simulink model "w2_warplab_buffers"  (Simulink 7.7)
settings: Solver=VariableStepDiscrete  SolverMode=SingleTasking  StartTime=0.0  StopTime=200000  RelTol=1e-3
InitFcn:
  | w2_warplab_buffers_init
StartFcn:
  | w2_warplab_buffers_init
values from neighbouring files (symbols this model uses):
  NumSamps_Rx_IQ = 2^14    (= 16384)    [w2_warplab_buffers_init.m]
  NumSamps_Rx_RSSI = 2^12    (= 4096)    [w2_warplab_buffers_init.m]
  NumSamps_Tx_IQ = 2^14    (= 16384)    [w2_warplab_buffers_init.m]
undefined symbols (not defined in the file or in its folder): gcbh, xlBlockLoadCallback, xlGetNormalizedPeriod
libraries: xbsIndex_r4 x752
(part 5 of 7)

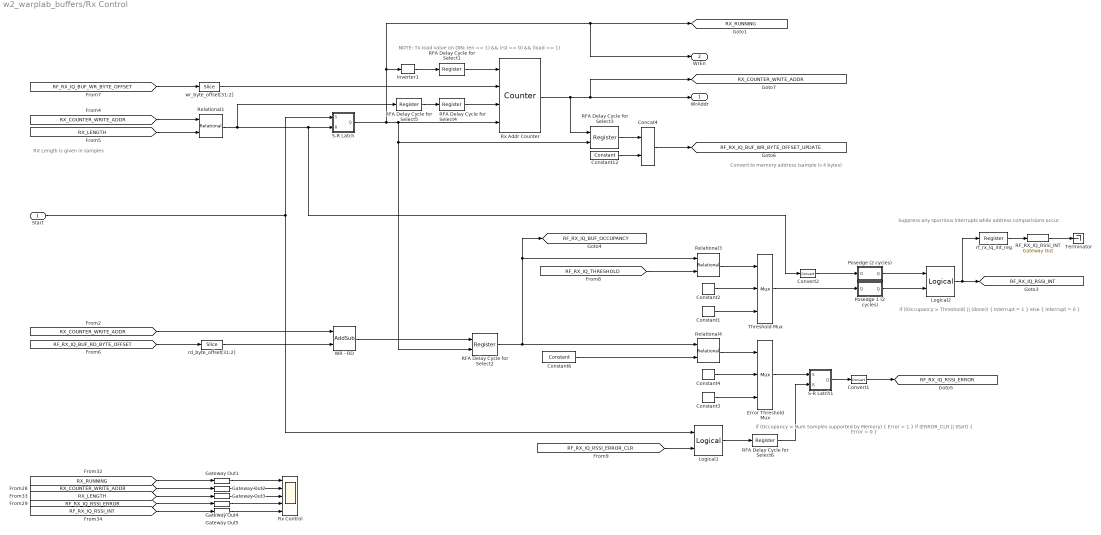
== system w2_warplab_buffers/Rx Control ==
  note: if ((Occupancy > Threshold) || (done)) {
      |     Interrupt = 1
      | } else {
      |     Interrupt = 0
      | }
  note: NOTE: To load value on DIN: (en == 1) && (rst == 0) && (load == 1)
  note: if (Occupancy > Num Samples supported by Memory) {
      |     Error = 1
      | }
      |
      | if (ERROR_CLR || Start) {
      |     Error = 0
      | }
  note: RX Length is given in samples
  note: Convert to memory address (sample is 4 bytes)
  note: Suppress any spurrious interrupts while
      | address comparisions occur.
  Start : Inport
  Concat4 : xbsIndex_r4/Concat  num_inputs=2  dbl_ovrd=off  block_type=concat
  Constant1 : xbsIndex_r4/Constant  const=1  gui_display_data_type=Fixed-point  arith_type=Unsigned  n_bits=1  bin_pt=0  preci_type=Single  exp_width=8  frac_width=24  explicit_period=off  period=1  equ=P=C  opselect=C  inp2=PCIN>>17  opr=+  inp1=P  carry=CIN  dbl_ovrd=off  block_type=constant
      settings: block_version=10.1.2
  Constant12 : xbsIndex_r4/Constant  const=0  gui_display_data_type=Fixed-point  arith_type=Unsigned  n_bits=2  bin_pt=0  preci_type=Single  exp_width=8  frac_width=24  explicit_period=off  period=1  equ=P=C  opselect=C  inp2=PCIN>>17  opr=+  inp1=P  carry=CIN  dbl_ovrd=off  block_type=constant
  Constant2 : xbsIndex_r4/Constant  const=0  gui_display_data_type=Fixed-point  arith_type=Unsigned  n_bits=1  bin_pt=0  preci_type=Single  exp_width=8  frac_width=24  explicit_period=off  period=1  equ=P=C  opselect=C  inp2=PCIN>>17  opr=+  inp1=P  carry=CIN  dbl_ovrd=off  block_type=constant
      settings: block_version=10.1.2
  Constant3 : xbsIndex_r4/Constant  const=1  gui_display_data_type=Fixed-point  arith_type=Unsigned  n_bits=1  bin_pt=0  preci_type=Single  exp_width=8  frac_width=24  explicit_period=off  period=1  equ=P=C  opselect=C  inp2=PCIN>>17  opr=+  inp1=P  carry=CIN  dbl_ovrd=off  block_type=constant
      settings: block_version=10.1.2
  Constant4 : xbsIndex_r4/Constant  const=0  gui_display_data_type=Fixed-point  arith_type=Unsigned  n_bits=1  bin_pt=0  preci_type=Single  exp_width=8  frac_width=24  explicit_period=off  period=1  equ=P=C  opselect=C  inp2=PCIN>>17  opr=+  inp1=P  carry=CIN  dbl_ovrd=off  block_type=constant
      settings: block_version=10.1.2
  Constant6 : xbsIndex_r4/Constant  const=NumSamps_Rx_IQ  gui_display_data_type=Fixed-point  arith_type=Unsigned  n_bits=30  bin_pt=0  preci_type=Single  exp_width=8  frac_width=24  explicit_period=off  period=1  equ=P=C  opselect=C  inp2=PCIN>>17  opr=+  inp1=P  carry=CIN  dbl_ovrd=off  block_type=constant
      settings: block_version=10.1.2
  Convert1 : xbsIndex_r4/Convert  gui_display_data_type=Fixed-point  arith_type=Unsigned  n_bits=1  bin_pt=0  float_type=Single  exp_bits=8  fraction_bits=24  quantization=Truncate  overflow=Wrap  en=off  latency=0  dbl_ovrd=off  pipeline=off  block_type=convert
      settings: block_version=10.1.2
  Convert2 : xbsIndex_r4/Convert  gui_display_data_type=Fixed-point  arith_type=Unsigned  n_bits=1  bin_pt=0  float_type=Single  exp_bits=8  fraction_bits=24  quantization=Truncate  overflow=Wrap  en=off  latency=0  dbl_ovrd=off  pipeline=off  block_type=convert
      settings: block_version=10.1.2
  Error Threshold Mux : xbsIndex_r4/Mux  inputs=2  en=off  latency=0  precision=Full  arith_type=Unsigned  n_bits=16  bin_pt=14  quantization=Truncate  overflow=Wrap  dbl_ovrd=off  block_type=mux
  Gateway Out{1..5} (5 alike) : xbsIndex_r4/Gateway Out  inherit_from_input=off  hdl_port=off  timing_constraint=None  locs_specified=off  LOCs={}  UseAsDAC=off  DACChannel='1'  block_type=gatewayout
      settings: infoedit="Gateway out block.  Converts Xilinx fixed point inputs into ouputs of type Simulink integer, double, or fixed point.<P><P>Hardware notes:  In hardware these blocks become top level output ports or are discarded, depending on how they are configured."  block_version=10.1.2
  Inverter1 : xbsIndex_r4/Inverter  en=off  latency=0  dbl_ovrd=off  block_type=inv
      settings: block_version=8.2
  Logical1 : xbsIndex_r4/Logical  logical_function=OR  inputs=2  en=off  latency=0  precision=Full  arith_type=Unsigned  n_bits=16  bin_pt=0  align_bp=on  dbl_ovrd=off  block_type=logical
  Logical2 : xbsIndex_r4/Logical  logical_function=OR  inputs=2  en=off  latency=0  precision=Full  arith_type=Unsigned  n_bits=16  bin_pt=0  align_bp=on  dbl_ovrd=off  block_type=logical
  Posedge (2 cycles) : Subsystem
  Posedge 1 (2 cycles) : Subsystem
  RFA Delay Cycle for Select{1,4..6} (4 alike) : xbsIndex_r4/Register  init=0  rst=off  en=off  dbl_ovrd=off  block_type=register
  RFA Delay Cycle for Select2 : xbsIndex_r4/Register  init=0  rst=off  en=on  dbl_ovrd=off  block_type=register
  RFA Delay Cycle for Select3 : xbsIndex_r4/Register  init=0  rst=off  en=on  dbl_ovrd=off  block_type=register
  RF_RX_IQ_RSSI_INT : xbsIndex_r4/Gateway Out  inherit_from_input=off  hdl_port=on  timing_constraint=None  locs_specified=off  LOCs={}  UseAsDAC=off  DACChannel='1'  block_type=gatewayout
      settings: block_version=8.2
  Relational1 : xbsIndex_r4/Relational  mode=a>=b  en=off  latency=0  dbl_ovrd=off  block_type=relational
      settings: block_version=8.2
  Relational3 : xbsIndex_r4/Relational  mode=a>b  en=off  latency=0  dbl_ovrd=off  block_type=relational
      settings: block_version=8.2
  Relational4 : xbsIndex_r4/Relational  mode=a>b  en=off  latency=0  dbl_ovrd=off  block_type=relational
      settings: block_version=8.2
  Rx Addr Counter : xbsIndex_r4/Counter  cnt_type=Free Running  cnt_to=Inf  operation=Up  start_count=0  cnt_by_val=1  arith_type=Unsigned  n_bits=30  bin_pt=0  load_pin=on  rst=on  en=on  explicit_period=off  period=1  dbl_ovrd=off  use_behavioral_HDL=off  implementation=Fabric  use_rpm=off  block_type=counter
      settings: block_version=8.2
  Rx Control : Scope  NumInputPorts=5
      settings: TimeRange=70000  YMin=0~0~0~0~0  YMax=1~1~1~100~20000
  S-R Latch : Subsystem
  S-R Latch1 : Subsystem
  Terminator : Terminator
  Threshold Mux : xbsIndex_r4/Mux  inputs=2  en=off  latency=0  precision=Full  arith_type=Unsigned  n_bits=16  bin_pt=14  quantization=Truncate  overflow=Wrap  dbl_ovrd=off  block_type=mux
  WR - RD : xbsIndex_r4/AddSub  mode=Subtraction  use_carryin=off  use_carryout=off  en=off  latency=0  precision=User Defined  arith_type=Unsigned  n_bits=30  bin_pt=0  quantization=Truncate  overflow=Wrap  dbl_ovrd=off  use_behavioral_HDL=off  hw_selection=Fabric  pipelined=off  block_type=addsub
  rd_byte_offset[31:2] : xbsIndex_r4/Slice  nbits=30  boolean_output=off  mode=Lower Bit Location + Width  bit1=0  base1=MSB of Input  bit0=2  base0=LSB of Input  dbl_ovrd=off  block_type=slice
  rf_rx_iq_int_reg : xbsIndex_r4/Register  init=0  rst=off  en=off  dbl_ovrd=off  block_type=register
  wr_byte_offset[31:2] : xbsIndex_r4/Slice  nbits=30  boolean_output=off  mode=Lower Bit Location + Width  bit1=0  base1=MSB of Input  bit0=2  base0=LSB of Input  dbl_ovrd=off  block_type=slice
  WrAddr : Outport
  WrEn : Outport  Port=2
  tag scope: RF_RX_IQ_BUF_OCCUPANCY=global, RF_RX_IQ_BUF_WR_BYTE_OFFSET_UPDATE=global, RF_RX_IQ_RSSI_ERROR=global, RF_RX_IQ_RSSI_INT=global, RX_COUNTER_WRITE_ADDR=global, RX_RUNNING=global
  wires:
  S-R Latch/1(Q) -> Inverter1/1, WrEn/1, [RX_RUNNING], Rx Addr Counter/4, RFA Delay Cycle for Select3/2, RFA Delay Cycle for Select2/2
  Gateway Out5/1 -> Rx Control/5
  Gateway Out4/1 -> Rx Control/4
  Gateway Out3/1 -> Rx Control/3
  Gateway Out2/1 -> Rx Control/2
  Gateway Out1/1 -> Rx Control/1
  [RF_RX_IQ_BUF_RD_BYTE_OFFSET] -> rd_byte_offset[31:2]/1
  Relational3/1 -> Threshold Mux/1
  Constant1/1 -> Threshold Mux/3
  Constant2/1 -> Threshold Mux/2
  [RF_RX_IQ_THRESHOLD] -> Relational3/2
  Relational4/1 -> Error Threshold Mux/1
  Constant3/1 -> Error Threshold Mux/3
  Constant4/1 -> Error Threshold Mux/2
  Error Threshold Mux/1 -> S-R Latch1/1(S)
  Constant6/1 -> Relational4/2
  [RX_LENGTH] -> Relational1/2
  Relational1/1 -> RFA Delay Cycle for Select5/1, S-R Latch/2(R), Convert2/1
  Rx Addr Counter/1 -> [RX_COUNTER_WRITE_ADDR], WrAddr/1, RFA Delay Cycle for Select3/1
  Constant12/1 -> Concat4/2
  Concat4/1 -> [RF_RX_IQ_BUF_WR_BYTE_OFFSET_UPDATE]
  S-R Latch1/1(Q) -> Convert1/1
  Convert1/1 -> [RF_RX_IQ_RSSI_ERROR]
  [RF_RX_IQ_BUF_WR_BYTE_OFFSET] -> wr_byte_offset[31:2]/1
  wr_byte_offset[31:2]/1 -> Rx Addr Counter/2
  Inverter1/1 -> RFA Delay Cycle for Select1/1
  RFA Delay Cycle for Select1/1 -> Rx Addr Counter/1
  RF_RX_IQ_RSSI_INT/1 -> Terminator/1
  Logical1/1 -> RFA Delay Cycle for Select6/1
  [RF_RX_IQ_RSSI_ERROR_CLR] -> Logical1/2
  RFA Delay Cycle for Select3/1 -> Concat4/1
  RFA Delay Cycle for Select4/1 -> Rx Addr Counter/3
  RFA Delay Cycle for Select5/1 -> RFA Delay Cycle for Select4/1
  Logical2/1 -> [RF_RX_IQ_RSSI_INT], rf_rx_iq_int_reg/1
  Threshold Mux/1 -> Posedge 1 (2 cycles)/1(D)
  Convert2/1 -> Posedge (2 cycles)/1(D)
  [RX_COUNTER_WRITE_ADDR] -> Relational1/1
  [RX_COUNTER_WRITE_ADDR] -> WR - RD/1
  rd_byte_offset[31:2]/1 -> WR - RD/2
  WR - RD/1 -> RFA Delay Cycle for Select2/1
  RFA Delay Cycle for Select2/1 -> Relational4/1, [RF_RX_IQ_BUF_OCCUPANCY], Relational3/1
  Start/1 -> S-R Latch/1(S), Logical1/1
  RFA Delay Cycle for Select6/1 -> S-R Latch1/2(R)
  [RX_RUNNING] -> Gateway Out1/1
  [RX_COUNTER_WRITE_ADDR] -> Gateway Out2/1
  [RX_LENGTH] -> Gateway Out3/1
  [RF_RX_IQ_RSSI_ERROR] -> Gateway Out4/1
  [RF_RX_IQ_RSSI_INT] -> Gateway Out5/1
  Posedge 1 (2 cycles)/1(Q) -> Logical2/2
  Posedge (2 cycles)/1(Q) -> Logical2/1
  rf_rx_iq_int_reg/1 -> RF_RX_IQ_RSSI_INT/1

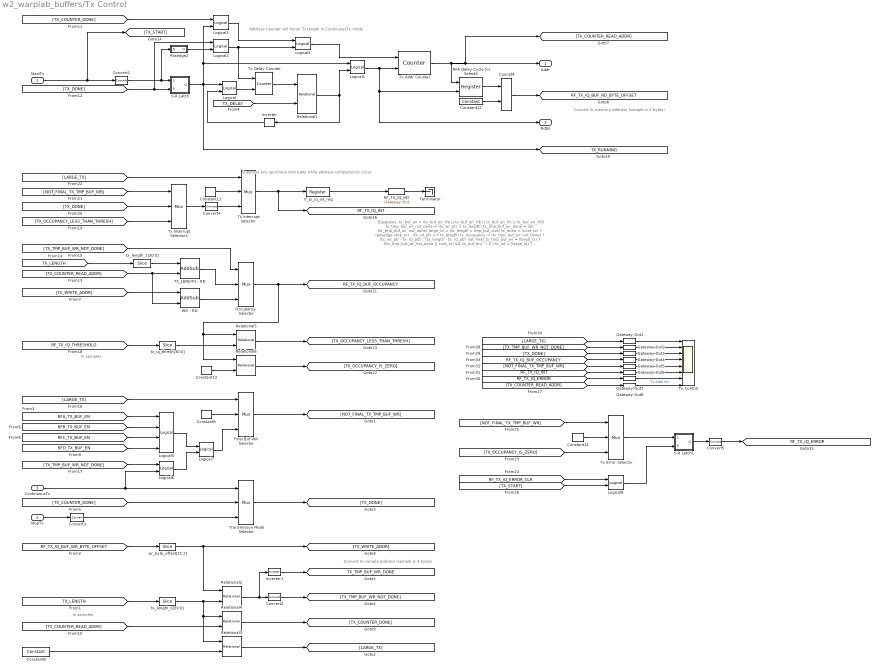
== system w2_warplab_buffers/Tx Control ==
  note: Address Counter will honor TxLength in ContinuousTx mode
  note: Convert to memory address (sample is 4 bytes)
  note: Convert to sample address (sample is 4 bytes)
  note: Equations:
      |   tx_buf_en               = (tx_buf_en_rfa || tx_buf_en_rfb || tx_buf_en_rfc || tx_buf_en_rfd)
      |
      |   tx_tmp_buf_wr_not_done  = (tx_wr_ptr < tx_length)
      |
      |   tx_tmp_buf_wr_done      = not (tx_tmp_buf_wr_not_done)
      |
      |   large_tx                = (tx_length > tmp_buf_size)
      |
      |   tx_done                 = (cont_tx) ? (posedge stop_tx) : (tx_rd_ptr >= tx_length)
      |
      |   tx_occupancy            = (tx_tmp_buf_wr_not_done) ? (tx_wr_ptr - tx_rd_ptr) : (tx_length - tx_rd_ptr)
      |
      |   not_final_tx_tmp_buf_wr = (large_tx) ? ((tx_tmp_buf_wr_not_done || cont_tx) && tx_buf_en) : ( 0 )
      |
      |   tx_int                  = (large_tx) ? ((not_final_tx_tmp_buf_wr) ? (tx_occupancy < tx_threshold) : tx_done) : ( 0 )
      |
      |   tx_err                  = (not_final_tx_tmp_buf_wr) ? (tx_occupancy == 0) : (0)
  note: In samples
  note: In samples
  note: Suppress any spurrious interrupts while
      | address comparisions occur.
  StartTx : Inport
  StopTx : Inport  Port=2
  ContinuousTx : Inport  Port=3
  Concat4 : xbsIndex_r4/Concat  num_inputs=2  dbl_ovrd=off  block_type=concat
  Constant11 : xbsIndex_r4/Constant  const=0  gui_display_data_type=Fixed-point  arith_type=Unsigned  n_bits=1  bin_pt=0  preci_type=Single  exp_width=8  frac_width=24  explicit_period=off  period=1  equ=P=C  opselect=C  inp2=PCIN>>17  opr=+  inp1=P  carry=CIN  dbl_ovrd=off  block_type=constant
      settings: block_version=10.1.2
  Constant12 : xbsIndex_r4/Constant  const=0  gui_display_data_type=Fixed-point  arith_type=Unsigned  n_bits=2  bin_pt=0  preci_type=Single  exp_width=8  frac_width=24  explicit_period=off  period=1  equ=P=C  opselect=C  inp2=PCIN>>17  opr=+  inp1=P  carry=CIN  dbl_ovrd=off  block_type=constant
  Constant13 : xbsIndex_r4/Constant  const=0  gui_display_data_type=Fixed-point  arith_type=Unsigned  n_bits=30  bin_pt=0  preci_type=Single  exp_width=8  frac_width=24  explicit_period=off  period=1  equ=P=C  opselect=C  inp2=PCIN>>17  opr=+  inp1=P  carry=CIN  dbl_ovrd=off  block_type=constant
      settings: block_version=10.1.2
  Constant14 : xbsIndex_r4/Constant  const=0  gui_display_data_type=Boolean  arith_type=Boolean  n_bits=1  bin_pt=0  preci_type=Single  exp_width=8  frac_width=24  explicit_period=off  period=1  equ=P=C  opselect=C  inp2=PCIN>>17  opr=+  inp1=P  carry=CIN  dbl_ovrd=off  block_type=constant
      settings: block_version=10.1.2
  Constant8 : xbsIndex_r4/Constant  const=NumSamps_Tx_IQ  gui_display_data_type=Fixed-point  arith_type=Unsigned  n_bits=30  bin_pt=0  preci_type=Single  exp_width=8  frac_width=24  explicit_period=off  period=1  equ=P=C  opselect=C  inp2=PCIN>>17  opr=+  inp1=P  carry=CIN  dbl_ovrd=off  block_type=constant
      settings: block_version=10.1.2
  Constant9 : xbsIndex_r4/Constant  const=0  gui_display_data_type=Fixed-point  arith_type=Unsigned  n_bits=1  bin_pt=0  preci_type=Single  exp_width=8  frac_width=24  explicit_period=off  period=1  equ=P=C  opselect=C  inp2=PCIN>>17  opr=+  inp1=P  carry=CIN  dbl_ovrd=off  block_type=constant
      settings: block_version=10.1.2
  Convert1 : xbsIndex_r4/Convert  gui_display_data_type=Fixed-point  arith_type=Boolean  n_bits=1  bin_pt=0  float_type=Single  exp_bits=8  fraction_bits=24  quantization=Truncate  overflow=Wrap  en=off  latency=0  dbl_ovrd=off  pipeline=off  block_type=convert
  Convert2 : xbsIndex_r4/Convert  gui_display_data_type=Fixed-point  arith_type=Unsigned  n_bits=1  bin_pt=0  float_type=Single  exp_bits=8  fraction_bits=24  quantization=Truncate  overflow=Wrap  en=off  latency=0  dbl_ovrd=off  pipeline=off  block_type=convert
  Convert3 : xbsIndex_r4/Convert  gui_display_data_type=Fixed-point  arith_type=Boolean  n_bits=1  bin_pt=0  float_type=Single  exp_bits=8  fraction_bits=24  quantization=Truncate  overflow=Wrap  en=off  latency=0  dbl_ovrd=off  pipeline=off  block_type=convert
  Convert4 : xbsIndex_r4/Convert  gui_display_data_type=Fixed-point  arith_type=Unsigned  n_bits=1  bin_pt=0  float_type=Single  exp_bits=8  fraction_bits=24  quantization=Truncate  overflow=Wrap  en=off  latency=0  dbl_ovrd=off  pipeline=off  block_type=convert
  Convert5 : xbsIndex_r4/Convert  gui_display_data_type=Fixed-point  arith_type=Unsigned  n_bits=1  bin_pt=0  float_type=Single  exp_bits=8  fraction_bits=24  quantization=Truncate  overflow=Wrap  en=off  latency=0  dbl_ovrd=off  pipeline=off  block_type=convert
      settings: block_version=10.1.2
  Final Buf WR  Selector : xbsIndex_r4/Mux  inputs=2  en=off  latency=0  precision=Full  arith_type=Unsigned  n_bits=16  bin_pt=14  quantization=Truncate  overflow=Wrap  dbl_ovrd=off  block_type=mux
      settings: block_version=9.1.01
  Gateway Out{1..8} (8 alike) : xbsIndex_r4/Gateway Out  inherit_from_input=off  hdl_port=off  timing_constraint=None  locs_specified=off  LOCs={}  UseAsDAC=off  DACChannel='1'  block_type=gatewayout
      settings: infoedit="Gateway out block.  Converts Xilinx fixed point inputs into ouputs of type Simulink integer, double, or fixed point.<P><P>Hardware notes:  In hardware these blocks become top level output ports or are discarded, depending on how they are configured."  block_version=10.1.2
  Inverter : xbsIndex_r4/Inverter  en=off  latency=0  dbl_ovrd=off  block_type=inv
      settings: block_version=8.2
  Inverter1 : xbsIndex_r4/Inverter  en=off  latency=0  dbl_ovrd=off  block_type=inv
      settings: block_version=8.2
  Logical{,1,3,7} (4 alike) : xbsIndex_r4/Logical  logical_function=AND  inputs=2  en=off  latency=0  precision=Full  arith_type=Unsigned  n_bits=16  bin_pt=0  align_bp=on  dbl_ovrd=off  block_type=logical
      settings: block_version=8.2
  Logical{2,4,6,8} (4 alike) : xbsIndex_r4/Logical  logical_function=OR  inputs=2  en=off  latency=0  precision=Full  arith_type=Unsigned  n_bits=16  bin_pt=0  align_bp=on  dbl_ovrd=off  block_type=logical
      Logical2 settings: block_version=8.2
      Logical6 settings: block_version=8.2
      Logical8 settings: block_version=8.2
  Logical5 : xbsIndex_r4/Logical  logical_function=OR  inputs=4  en=off  latency=0  precision=Full  arith_type=Unsigned  n_bits=16  bin_pt=0  align_bp=on  dbl_ovrd=off  block_type=logical
      settings: block_version=8.2
  Occupancy  Selector : xbsIndex_r4/Mux  inputs=2  en=off  latency=0  precision=Full  arith_type=Unsigned  n_bits=16  bin_pt=14  quantization=Truncate  overflow=Wrap  dbl_ovrd=off  block_type=mux
      settings: block_version=9.1.01
  Posedge2 : Subsystem
  RFA Delay Cycle for Select3 : xbsIndex_r4/Register  init=0  rst=off  en=on  dbl_ovrd=off  block_type=register
  RF_TX_IQ_INT : xbsIndex_r4/Gateway Out  inherit_from_input=off  hdl_port=on  timing_constraint=None  locs_specified=off  LOCs={}  UseAsDAC=off  DACChannel='1'  block_type=gatewayout
      settings: block_version=8.2
  Relational1 : xbsIndex_r4/Relational  mode=a>=b  en=off  latency=0  dbl_ovrd=off  block_type=relational
      settings: block_version=8.2
  Relational2 : xbsIndex_r4/Relational  mode=a<b  en=off  latency=0  dbl_ovrd=off  block_type=relational
      settings: block_version=8.2
  Relational3 : xbsIndex_r4/Relational  mode=a>b  en=off  latency=0  dbl_ovrd=off  block_type=relational
      settings: block_version=8.2
  Relational4 : xbsIndex_r4/Relational  mode=a<=b  en=off  latency=0  dbl_ovrd=off  block_type=relational
      settings: block_version=8.2
  Relational5 : xbsIndex_r4/Relational  mode=a<b  en=off  latency=0  dbl_ovrd=off  block_type=relational
      settings: block_version=8.2
  Relational6 : xbsIndex_r4/Relational  mode=a=b  en=off  latency=0  dbl_ovrd=off  block_type=relational
      settings: block_version=8.2
  S-R Latch : Subsystem
  S-R Latch1 : Subsystem
  TX_LENGTH - RD : xbsIndex_r4/AddSub  mode=Subtraction  use_carryin=off  use_carryout=off  en=off  latency=0  precision=User Defined  arith_type=Unsigned  n_bits=30  bin_pt=0  quantization=Truncate  overflow=Saturate  dbl_ovrd=off  use_behavioral_HDL=off  hw_selection=Fabric  pipelined=off  block_type=addsub
  Terminator : Terminator
  Transmisson Mode Selector : xbsIndex_r4/Mux  inputs=2  en=off  latency=0  precision=Full  arith_type=Unsigned  n_bits=16  bin_pt=14  quantization=Truncate  overflow=Wrap  dbl_ovrd=off  block_type=mux
      settings: block_version=9.1.01
  Tx Addr Counter : xbsIndex_r4/Counter  cnt_type=Free Running  cnt_to=Inf  operation=Up  start_count=0  cnt_by_val=1  arith_type=Unsigned  n_bits=30  bin_pt=0  load_pin=off  rst=on  en=on  explicit_period=off  period=1  dbl_ovrd=off  use_behavioral_HDL=off  implementation=Fabric  use_rpm=off  block_type=counter
      settings: block_version=8.2
  Tx Control : Scope  NumInputPorts=8
      settings: TimeRange=70000  YMin=0~0~0~0~0~0~0~0  YMax=2~1~1~1~1~100~1~20000  SaveName=ScopeData3
  Tx Delay Counter : xbsIndex_r4/Counter  cnt_type=Free Running  cnt_to=Inf  operation=Up  start_count=0  cnt_by_val=1  arith_type=Unsigned  n_bits=32  bin_pt=0  load_pin=off  rst=on  en=on  explicit_period=off  period=1  dbl_ovrd=off  use_behavioral_HDL=off  implementation=Fabric  use_rpm=off  block_type=counter
      settings: block_version=8.2
  Tx Error Selector : xbsIndex_r4/Mux  inputs=2  en=off  latency=0  precision=Full  arith_type=Unsigned  n_bits=16  bin_pt=14  quantization=Truncate  overflow=Wrap  dbl_ovrd=off  block_type=mux
      settings: block_version=9.1.01
  Tx Interrupt Selector : xbsIndex_r4/Mux  inputs=2  en=off  latency=0  precision=Full  arith_type=Unsigned  n_bits=16  bin_pt=14  quantization=Truncate  overflow=Wrap  dbl_ovrd=off  block_type=mux
      settings: block_version=9.1.01
  Tx Interrupt Selector1 : xbsIndex_r4/Mux  inputs=2  en=off  latency=0  precision=Full  arith_type=Unsigned  n_bits=16  bin_pt=14  quantization=Truncate  overflow=Wrap  dbl_ovrd=off  block_type=mux
      settings: block_version=9.1.01
  WR - RD : xbsIndex_r4/AddSub  mode=Subtraction  use_carryin=off  use_carryout=off  en=off  latency=0  precision=User Defined  arith_type=Unsigned  n_bits=30  bin_pt=0  quantization=Truncate  overflow=Saturate  dbl_ovrd=off  use_behavioral_HDL=off  hw_selection=Fabric  pipelined=off  block_type=addsub
  rf_tx_iq_int_reg : xbsIndex_r4/Register  init=0  rst=off  en=off  dbl_ovrd=off  block_type=register
  tx_iq_thresh[30:0] : xbsIndex_r4/Slice  nbits=30  boolean_output=off  mode=Lower Bit Location + Width  bit1=0  base1=MSB of Input  bit0=0  base0=LSB of Input  dbl_ovrd=off  block_type=slice
  tx_length_0[30:0] : xbsIndex_r4/Slice  nbits=30  boolean_output=off  mode=Lower Bit Location + Width  bit1=0  base1=MSB of Input  bit0=0  base0=LSB of Input  dbl_ovrd=off  block_type=slice
  tx_length_1[30:0] : xbsIndex_r4/Slice  nbits=30  boolean_output=off  mode=Lower Bit Location + Width  bit1=0  base1=MSB of Input  bit0=0  base0=LSB of Input  dbl_ovrd=off  block_type=slice
  wr_byte_offset[31:2] : xbsIndex_r4/Slice  nbits=30  boolean_output=off  mode=Lower Bit Location + Width  bit1=0  base1=MSB of Input  bit0=2  base0=LSB of Input  dbl_ovrd=off  block_type=slice
  Addr : Outport
  RdEn : Outport  Port=2
  tag scope: RF_TX_IQ_BUF_OCCUPANCY=global, RF_TX_IQ_BUF_RD_BYTE_OFFSET=global, RF_TX_IQ_ERROR=global, RF_TX_IQ_INT=global, TX_RUNNING=global, TX_TMP_BUF_WR_DONE=global
  wires:
  Tx Delay Counter/1 -> Relational1/1
  [TX_DELAY] -> Relational1/2
  StartTx/1 -> Convert1/1, [TX_START]
  Logical/1 -> Tx Delay Counter/2
  S-R Latch/1(Q) -> Logical/1, Logical1/1, Logical3/2, [TX_RUNNING]
  Relational1/1 -> Inverter/1, Logical1/2
  Inverter/1 -> Logical/2
  Logical1/1 -> Tx Addr Counter/2, RdEn/1, RFA Delay Cycle for Select3/2
  Tx Addr Counter/1 -> Addr/1, RFA Delay Cycle for Select3/1, [TX_COUNTER_READ_ADDR]
  Posedge2/1(Q) -> Logical2/2
  Logical2/1 -> Tx Delay Counter/1, Logical4/2
  Convert1/1 -> S-R Latch/1(S), Posedge2/1(D)
  Gateway Out5/1 -> Tx Control/5
  Gateway Out4/1 -> Tx Control/4
  Gateway Out3/1 -> Tx Control/3
  Gateway Out2/1 -> Tx Control/2
  Gateway Out1/1 -> Tx Control/1
  Gateway Out6/1 -> Tx Control/6
  Gateway Out7/1 -> Tx Control/7
  Gateway Out8/1 -> Tx Control/8  "Tx Addr Ctr"
  Logical3/1 -> Logical4/1
  Logical4/1 -> Tx Addr Counter/1
  Constant12/1 -> Concat4/2
  Concat4/1 -> [RF_TX_IQ_BUF_RD_BYTE_OFFSET]
  RFA Delay Cycle for Select3/1 -> Concat4/1
  [RF_TX_IQ_BUF_WR_BYTE_OFFSET] -> wr_byte_offset[31:2]/1
  wr_byte_offset[31:2]/1 -> Relational2/1, [TX_WRITE_ADDR]
  [TX_LENGTH] -> tx_length_0[30:0]/1
  Constant8/1 -> Relational3/2
  Relational3/1 -> [LARGE_TX]
  Relational2/1 -> Inverter1/1, Convert2/1
  Inverter1/1 -> [TX_TMP_BUF_WR_DONE]
  [TX_COUNTER_READ_ADDR] -> Relational4/2
  Relational4/1 -> [TX_COUNTER_DONE]
  [TX_COUNTER_DONE] -> Logical3/1
  ContinuousTx/1 -> Transmisson Mode Selector/1, Logical6/2
  StopTx/1 -> Convert3/1
  Convert3/1 -> Transmisson Mode Selector/3
  [TX_COUNTER_DONE] -> Transmisson Mode Selector/2
  Transmisson Mode Selector/1 -> [TX_DONE]
  [TX_DONE] -> S-R Latch/2(R), Logical2/1
  [TX_TMP_BUF_WR_NOT_DONE] -> Occupancy  Selector/1
  Occupancy  Selector/1 -> [RF_TX_IQ_BUF_OCCUPANCY], Relational5/1, Relational6/1
  [LARGE_TX] -> Final Buf WR  Selector/1
  [TX_LENGTH] -> tx_length_1[30:0]/1
  [TX_COUNTER_READ_ADDR] -> TX_LENGTH - RD/2, WR - RD/2
  [TX_WRITE_ADDR] -> WR - RD/1
  TX_LENGTH - RD/1 -> Occupancy  Selector/2
  WR - RD/1 -> Occupancy  Selector/3
  Constant9/1 -> Final Buf WR  Selector/2
  [TX_TMP_BUF_WR_NOT_DONE] -> Logical6/1
  [RFA_TX_BUF_EN] -> Logical5/1
  [RFB_TX_BUF_EN] -> Logical5/2
  [RFC_TX_BUF_EN] -> Logical5/3
  [RFD_TX_BUF_EN] -> Logical5/4
  Logical5/1 -> Logical7/1
  Logical6/1 -> Logical7/2
  Logical7/1 -> Final Buf WR  Selector/3
  Constant11/1 -> Tx Interrupt Selector/2
  Final Buf WR  Selector/1 -> [NOT_FINAL_TX_TMP_BUF_WR]
  Constant13/1 -> Relational6/2
  [RF_TX_IQ_THRESHOLD] -> tx_iq_thresh[30:0]/1
  Relational6/1 -> [TX_OCCUPANCY_IS_ZERO]
  Relational5/1 -> [TX_OCCUPANCY_LESS_THAN_THRESH]
  RF_TX_IQ_INT/1 -> Terminator/1
  [NOT_FINAL_TX_TMP_BUF_WR] -> Tx Interrupt Selector1/1
  [TX_DONE] -> Tx Interrupt Selector1/2
  [TX_OCCUPANCY_LESS_THAN_THRESH] -> Tx Interrupt Selector1/3
  [LARGE_TX] -> Tx Interrupt Selector/1
  Tx Interrupt Selector1/1 -> Convert4/1
  Tx Interrupt Selector/1 -> [RF_TX_IQ_INT], rf_tx_iq_int_reg/1
  Convert2/1 -> [TX_TMP_BUF_WR_NOT_DONE]
  Convert4/1 -> Tx Interrupt Selector/3
  [NOT_FINAL_TX_TMP_BUF_WR] -> Tx Error Selector/1
  [TX_OCCUPANCY_IS_ZERO] -> Tx Error Selector/3
  Constant14/1 -> Tx Error Selector/2
  S-R Latch1/1(Q) -> Convert5/1
  Convert5/1 -> [RF_TX_IQ_ERROR]
  Tx Error Selector/1 -> S-R Latch1/1(S)
  [RF_TX_IQ_ERROR_CLR] -> Logical8/1
  Logical8/1 -> S-R Latch1/2(R)
  [TX_START] -> Logical8/2
  [TX_COUNTER_READ_ADDR] -> Gateway Out8/1
  [LARGE_TX] -> Gateway Out1/1
  [TX_TMP_BUF_WR_NOT_DONE] -> Gateway Out2/1
  [TX_DONE] -> Gateway Out3/1
  [RF_TX_IQ_BUF_OCCUPANCY] -> Gateway Out4/1
  [NOT_FINAL_TX_TMP_BUF_WR] -> Gateway Out5/1
  [RF_TX_IQ_INT] -> Gateway Out6/1
  [RF_TX_IQ_ERROR] -> Gateway Out7/1
  tx_length_0[30:0]/1 -> Relational2/2, Relational3/1, Relational4/1
  tx_iq_thresh[30:0]/1 -> Relational5/2
  tx_length_1[30:0]/1 -> TX_LENGTH - RD/1
  rf_tx_iq_int_reg/1 -> RF_TX_IQ_INT/1

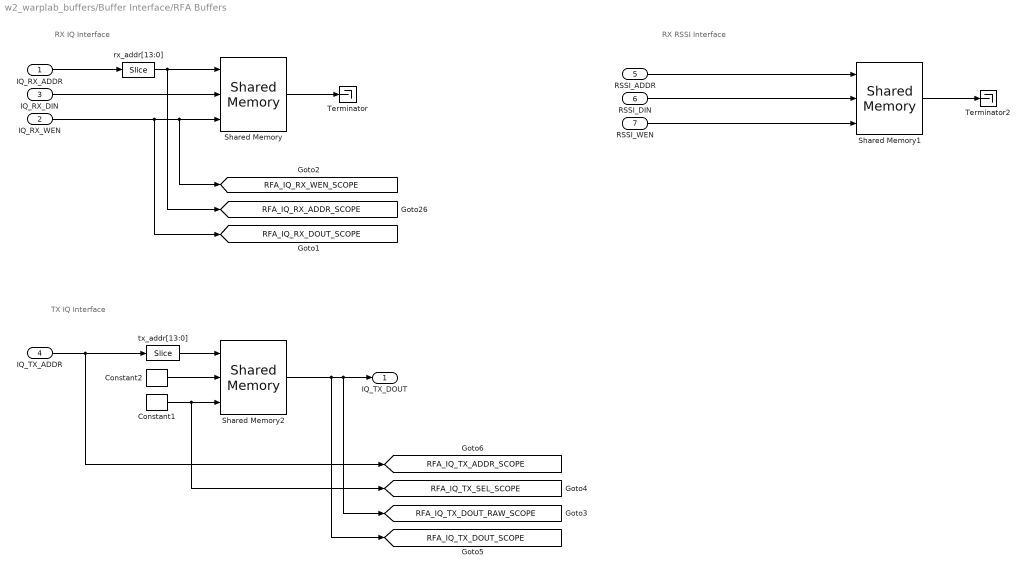
== system w2_warplab_buffers/Buffer Interface/RFA Buffers ==
  note: RX IQ Interface
  note: TX IQ Interface
  note: RX RSSI Interface
  IQ_RX_ADDR : Inport
  IQ_RX_WEN : Inport  Port=2
  IQ_RX_DIN : Inport  Port=3
  IQ_TX_ADDR : Inport  Port=4
  RSSI_ADDR : Inport  Port=5
  RSSI_DIN : Inport  Port=6
  RSSI_WEN : Inport  Port=7
  Constant1 : xbsIndex_r4/Constant  const=0  gui_display_data_type=Fixed-point  arith_type=Boolean  n_bits=32  bin_pt=0  preci_type=Single  exp_width=8  frac_width=24  explicit_period=off  period=1  equ=P=C  opselect=C  inp2=PCIN>>17  opr=+  inp1=P  carry=CIN  dbl_ovrd=off  block_type=constant
      settings: block_version=10.1.2
  Constant2 : xbsIndex_r4/Constant  const=0  gui_display_data_type=Fixed-point  arith_type=Unsigned  n_bits=32  bin_pt=0  preci_type=Single  exp_width=8  frac_width=24  explicit_period=off  period=1  equ=P=C  opselect=C  inp2=PCIN>>17  opr=+  inp1=P  carry=CIN  dbl_ovrd=off  block_type=constant
      settings: block_version=10.1.2
  Shared Memory : xbsIndex_r4/Shared Memory  shared_memory_name='RFA_IQ_Rx_Buffer'  depth=NumSamps_Rx_IQ  ownership=Locally Owned and Initialized  initVector=0  en=off  mutex=Unprotected  mode=Read and Write  write_mode=Read After Write  time_out=0  latency=1  explicit_data_type=on  gui_display_data_type=Fixed-point  arith_type=Unsigned  n_bits=32  bin_pt=0  preci_type=Single  implementation=Block RAM  use_rpm=off  block_type=shmem
      settings: AttributesFormatString=<< %<shared_memory_name> >>  block_version=10.1.2
  Shared Memory1 : xbsIndex_r4/Shared Memory  shared_memory_name='RFA_RSSI_Buffer'  depth=NumSamps_Rx_RSSI/2  ownership=Locally Owned and Initialized  initVector=0  en=off  mutex=Unprotected  mode=Read and Write  write_mode=Read After Write  time_out=0  latency=1  explicit_data_type=on  gui_display_data_type=Fixed-point  arith_type=Unsigned  n_bits=32  bin_pt=0  preci_type=Single  implementation=Block RAM  use_rpm=off  block_type=shmem
      settings: AttributesFormatString=<< %<shared_memory_name> >>  block_version=10.1.2
  Shared Memory2 : xbsIndex_r4/Shared Memory  shared_memory_name='RFA_IQ_Tx_Buffer'  depth=NumSamps_Tx_IQ  ownership=Locally Owned and Initialized  initVector=0  en=off  mutex=Unprotected  mode=Read and Write  write_mode=Read After Write  time_out=0  latency=1  explicit_data_type=on  gui_display_data_type=Fixed-point  arith_type=Unsigned  n_bits=32  bin_pt=0  preci_type=Single  implementation=Block RAM  use_rpm=off  block_type=shmem
      settings: AttributesFormatString=<< %<shared_memory_name> >>  block_version=10.1.2
  Terminator : Terminator
  Terminator2 : Terminator
  rx_addr[13:0] : xbsIndex_r4/Slice  nbits=14  boolean_output=off  mode=Lower Bit Location + Width  bit1=0  base1=MSB of Input  bit0=0  base0=LSB of Input  dbl_ovrd=off  block_type=slice
  tx_addr[13:0] : xbsIndex_r4/Slice  nbits=14  boolean_output=off  mode=Lower Bit Location + Width  bit1=0  base1=MSB of Input  bit0=0  base0=LSB of Input  dbl_ovrd=off  block_type=slice
  IQ_TX_DOUT : Outport
  tag scope: RFA_IQ_RX_ADDR_SCOPE=global, RFA_IQ_RX_DOUT_SCOPE=global, RFA_IQ_RX_WEN_SCOPE=global, RFA_IQ_TX_ADDR_SCOPE=global, RFA_IQ_TX_DOUT_RAW_SCOPE=global, RFA_IQ_TX_DOUT_SCOPE=global, RFA_IQ_TX_SEL_SCOPE=global
  wires:
  IQ_RX_WEN/1 -> Shared Memory/3, [RFA_IQ_RX_WEN_SCOPE], [RFA_IQ_RX_DOUT_SCOPE]
  IQ_RX_ADDR/1 -> rx_addr[13:0]/1
  Shared Memory/1 -> Terminator/1
  IQ_RX_DIN/1 -> Shared Memory/2
  Shared Memory1/1 -> Terminator2/1
  RSSI_ADDR/1 -> Shared Memory1/1
  RSSI_DIN/1 -> Shared Memory1/2
  RSSI_WEN/1 -> Shared Memory1/3
  IQ_TX_ADDR/1 -> [RFA_IQ_TX_ADDR_SCOPE], tx_addr[13:0]/1
  Constant1/1 -> Shared Memory2/3, [RFA_IQ_TX_SEL_SCOPE]
  Constant2/1 -> Shared Memory2/2
  Shared Memory2/1 -> IQ_TX_DOUT/1, [RFA_IQ_TX_DOUT_RAW_SCOPE], [RFA_IQ_TX_DOUT_SCOPE]
  tx_addr[13:0]/1 -> Shared Memory2/1
  rx_addr[13:0]/1 -> Shared Memory/1, [RFA_IQ_RX_ADDR_SCOPE]

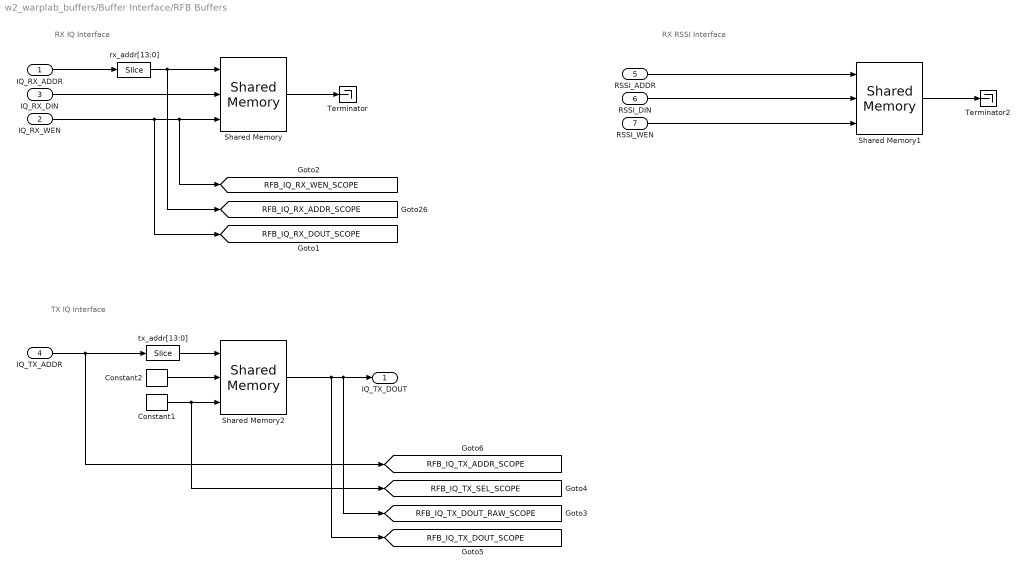
== system w2_warplab_buffers/Buffer Interface/RFB Buffers ==
  note: RX IQ Interface
  note: TX IQ Interface
  note: RX RSSI Interface
  IQ_RX_ADDR : Inport
  IQ_RX_WEN : Inport  Port=2
  IQ_RX_DIN : Inport  Port=3
  IQ_TX_ADDR : Inport  Port=4
  RSSI_ADDR : Inport  Port=5
  RSSI_DIN : Inport  Port=6
  RSSI_WEN : Inport  Port=7
  Constant1 : xbsIndex_r4/Constant  const=0  gui_display_data_type=Fixed-point  arith_type=Boolean  n_bits=32  bin_pt=0  preci_type=Single  exp_width=8  frac_width=24  explicit_period=off  period=1  equ=P=C  opselect=C  inp2=PCIN>>17  opr=+  inp1=P  carry=CIN  dbl_ovrd=off  block_type=constant
      settings: block_version=10.1.2
  Constant2 : xbsIndex_r4/Constant  const=0  gui_display_data_type=Fixed-point  arith_type=Unsigned  n_bits=32  bin_pt=0  preci_type=Single  exp_width=8  frac_width=24  explicit_period=off  period=1  equ=P=C  opselect=C  inp2=PCIN>>17  opr=+  inp1=P  carry=CIN  dbl_ovrd=off  block_type=constant
      settings: block_version=10.1.2
  Shared Memory : xbsIndex_r4/Shared Memory  shared_memory_name='RFB_IQ_Rx_Buffer'  depth=NumSamps_Rx_IQ  ownership=Locally Owned and Initialized  initVector=0  en=off  mutex=Unprotected  mode=Read and Write  write_mode=Read After Write  time_out=0  latency=1  explicit_data_type=on  gui_display_data_type=Fixed-point  arith_type=Unsigned  n_bits=32  bin_pt=0  preci_type=Single  implementation=Block RAM  use_rpm=off  block_type=shmem
      settings: AttributesFormatString=<< %<shared_memory_name> >>  block_version=10.1.2
  Shared Memory1 : xbsIndex_r4/Shared Memory  shared_memory_name='RFB_RSSI_Buffer'  depth=NumSamps_Rx_RSSI/2  ownership=Locally Owned and Initialized  initVector=0  en=off  mutex=Unprotected  mode=Read and Write  write_mode=Read After Write  time_out=0  latency=1  explicit_data_type=on  gui_display_data_type=Fixed-point  arith_type=Unsigned  n_bits=32  bin_pt=0  preci_type=Single  implementation=Block RAM  use_rpm=off  block_type=shmem
      settings: AttributesFormatString=<< %<shared_memory_name> >>  block_version=10.1.2
  Shared Memory2 : xbsIndex_r4/Shared Memory  shared_memory_name='RFB_IQ_Tx_Buffer'  depth=NumSamps_Tx_IQ  ownership=Locally Owned and Initialized  initVector=0  en=off  mutex=Unprotected  mode=Read and Write  write_mode=Read After Write  time_out=0  latency=1  explicit_data_type=on  gui_display_data_type=Fixed-point  arith_type=Unsigned  n_bits=32  bin_pt=0  preci_type=Single  implementation=Block RAM  use_rpm=off  block_type=shmem
      settings: AttributesFormatString=<< %<shared_memory_name> >>  block_version=10.1.2
  Terminator : Terminator
  Terminator2 : Terminator
  rx_addr[13:0] : xbsIndex_r4/Slice  nbits=14  boolean_output=off  mode=Lower Bit Location + Width  bit1=0  base1=MSB of Input  bit0=0  base0=LSB of Input  dbl_ovrd=off  block_type=slice
  tx_addr[13:0] : xbsIndex_r4/Slice  nbits=14  boolean_output=off  mode=Lower Bit Location + Width  bit1=0  base1=MSB of Input  bit0=0  base0=LSB of Input  dbl_ovrd=off  block_type=slice
  IQ_TX_DOUT : Outport
  tag scope: RFB_IQ_RX_ADDR_SCOPE=global, RFB_IQ_RX_DOUT_SCOPE=global, RFB_IQ_RX_WEN_SCOPE=global, RFB_IQ_TX_ADDR_SCOPE=global, RFB_IQ_TX_DOUT_RAW_SCOPE=global, RFB_IQ_TX_DOUT_SCOPE=global, RFB_IQ_TX_SEL_SCOPE=global
  wires:
  IQ_RX_WEN/1 -> Shared Memory/3, [RFB_IQ_RX_WEN_SCOPE], [RFB_IQ_RX_DOUT_SCOPE]
  IQ_RX_ADDR/1 -> rx_addr[13:0]/1
  Shared Memory/1 -> Terminator/1
  IQ_RX_DIN/1 -> Shared Memory/2
  Shared Memory1/1 -> Terminator2/1
  RSSI_ADDR/1 -> Shared Memory1/1
  RSSI_DIN/1 -> Shared Memory1/2
  RSSI_WEN/1 -> Shared Memory1/3
  IQ_TX_ADDR/1 -> [RFB_IQ_TX_ADDR_SCOPE], tx_addr[13:0]/1
  Constant1/1 -> Shared Memory2/3, [RFB_IQ_TX_SEL_SCOPE]
  Constant2/1 -> Shared Memory2/2
  Shared Memory2/1 -> IQ_TX_DOUT/1, [RFB_IQ_TX_DOUT_RAW_SCOPE], [RFB_IQ_TX_DOUT_SCOPE]
  tx_addr[13:0]/1 -> Shared Memory2/1
  rx_addr[13:0]/1 -> Shared Memory/1, [RFB_IQ_RX_ADDR_SCOPE]

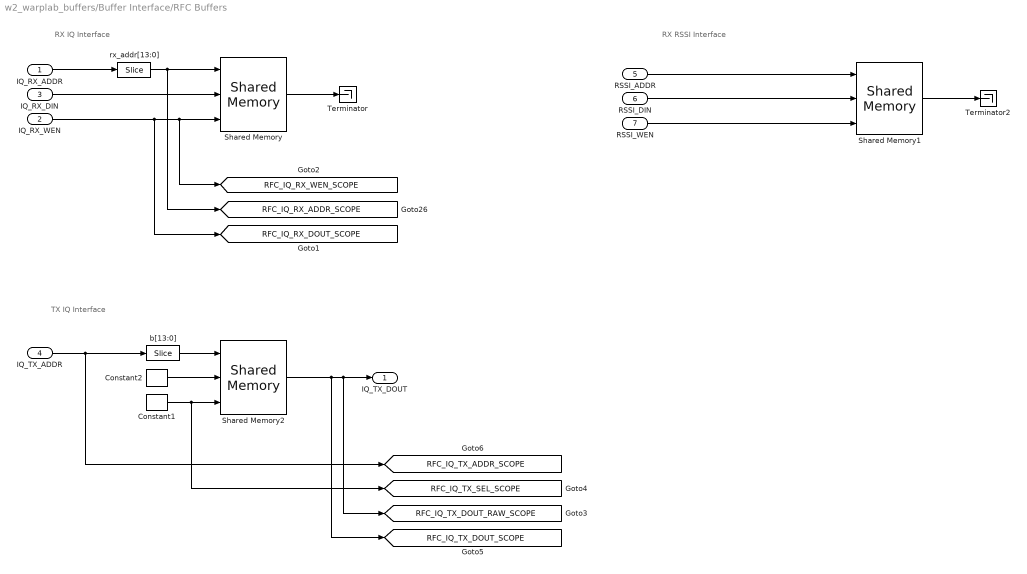
== system w2_warplab_buffers/Buffer Interface/RFC Buffers ==
  note: RX IQ Interface
  note: TX IQ Interface
  note: RX RSSI Interface
  IQ_RX_ADDR : Inport
  IQ_RX_WEN : Inport  Port=2
  IQ_RX_DIN : Inport  Port=3
  IQ_TX_ADDR : Inport  Port=4
  RSSI_ADDR : Inport  Port=5
  RSSI_DIN : Inport  Port=6
  RSSI_WEN : Inport  Port=7
  Constant1 : xbsIndex_r4/Constant  const=0  gui_display_data_type=Fixed-point  arith_type=Boolean  n_bits=32  bin_pt=0  preci_type=Single  exp_width=8  frac_width=24  explicit_period=off  period=1  equ=P=C  opselect=C  inp2=PCIN>>17  opr=+  inp1=P  carry=CIN  dbl_ovrd=off  block_type=constant
      settings: block_version=10.1.2
  Constant2 : xbsIndex_r4/Constant  const=0  gui_display_data_type=Fixed-point  arith_type=Unsigned  n_bits=32  bin_pt=0  preci_type=Single  exp_width=8  frac_width=24  explicit_period=off  period=1  equ=P=C  opselect=C  inp2=PCIN>>17  opr=+  inp1=P  carry=CIN  dbl_ovrd=off  block_type=constant
      settings: block_version=10.1.2
  Shared Memory : xbsIndex_r4/Shared Memory  shared_memory_name='RFC_IQ_Rx_Buffer'  depth=NumSamps_Rx_IQ  ownership=Locally Owned and Initialized  initVector=0  en=off  mutex=Unprotected  mode=Read and Write  write_mode=Read After Write  time_out=0  latency=1  explicit_data_type=on  gui_display_data_type=Fixed-point  arith_type=Unsigned  n_bits=32  bin_pt=0  preci_type=Single  implementation=Block RAM  use_rpm=off  block_type=shmem
      settings: AttributesFormatString=<< %<shared_memory_name> >>  block_version=10.1.2
  Shared Memory1 : xbsIndex_r4/Shared Memory  shared_memory_name='RFC_RSSI_Buffer'  depth=NumSamps_Rx_RSSI/2  ownership=Locally Owned and Initialized  initVector=0  en=off  mutex=Unprotected  mode=Read and Write  write_mode=Read After Write  time_out=0  latency=1  explicit_data_type=on  gui_display_data_type=Fixed-point  arith_type=Unsigned  n_bits=32  bin_pt=0  preci_type=Single  implementation=Block RAM  use_rpm=off  block_type=shmem
      settings: AttributesFormatString=<< %<shared_memory_name> >>  block_version=10.1.2
  Shared Memory2 : xbsIndex_r4/Shared Memory  shared_memory_name='RFC_IQ_Tx_Buffer'  depth=NumSamps_Tx_IQ  ownership=Locally Owned and Initialized  initVector=0  en=off  mutex=Unprotected  mode=Read and Write  write_mode=Read After Write  time_out=0  latency=1  explicit_data_type=on  gui_display_data_type=Fixed-point  arith_type=Unsigned  n_bits=32  bin_pt=0  preci_type=Single  implementation=Block RAM  use_rpm=off  block_type=shmem
      settings: AttributesFormatString=<< %<shared_memory_name> >>  block_version=10.1.2
  Terminator : Terminator
  Terminator2 : Terminator
  b[13:0] : xbsIndex_r4/Slice  nbits=14  boolean_output=off  mode=Lower Bit Location + Width  bit1=0  base1=MSB of Input  bit0=0  base0=LSB of Input  dbl_ovrd=off  block_type=slice
  rx_addr[13:0] : xbsIndex_r4/Slice  nbits=14  boolean_output=off  mode=Lower Bit Location + Width  bit1=0  base1=MSB of Input  bit0=0  base0=LSB of Input  dbl_ovrd=off  block_type=slice
  IQ_TX_DOUT : Outport
  tag scope: RFC_IQ_RX_ADDR_SCOPE=global, RFC_IQ_RX_DOUT_SCOPE=global, RFC_IQ_RX_WEN_SCOPE=global, RFC_IQ_TX_ADDR_SCOPE=global, RFC_IQ_TX_DOUT_RAW_SCOPE=global, RFC_IQ_TX_DOUT_SCOPE=global, RFC_IQ_TX_SEL_SCOPE=global
  wires:
  IQ_RX_WEN/1 -> Shared Memory/3, [RFC_IQ_RX_WEN_SCOPE], [RFC_IQ_RX_DOUT_SCOPE]
  IQ_RX_ADDR/1 -> rx_addr[13:0]/1
  Shared Memory/1 -> Terminator/1
  IQ_RX_DIN/1 -> Shared Memory/2
  Shared Memory1/1 -> Terminator2/1
  RSSI_ADDR/1 -> Shared Memory1/1
  RSSI_DIN/1 -> Shared Memory1/2
  RSSI_WEN/1 -> Shared Memory1/3
  IQ_TX_ADDR/1 -> [RFC_IQ_TX_ADDR_SCOPE], b[13:0]/1
  Constant1/1 -> Shared Memory2/3, [RFC_IQ_TX_SEL_SCOPE]
  Constant2/1 -> Shared Memory2/2
  Shared Memory2/1 -> IQ_TX_DOUT/1, [RFC_IQ_TX_DOUT_RAW_SCOPE], [RFC_IQ_TX_DOUT_SCOPE]
  b[13:0]/1 -> Shared Memory2/1
  rx_addr[13:0]/1 -> Shared Memory/1, [RFC_IQ_RX_ADDR_SCOPE]

== system w2_warplab_buffers/Buffer Interface/RFD Buffers ==
  note: RX IQ Interface
  note: TX IQ Interface
  note: RX RSSI Interface
  IQ_RX_ADDR : Inport
  IQ_RX_WEN : Inport  Port=2
  IQ_RX_DIN : Inport  Port=3
  IQ_TX_ADDR : Inport  Port=4
  RSSI_ADDR : Inport  Port=5
  RSSI_DIN : Inport  Port=6
  RSSI_WEN : Inport  Port=7
  Constant1 : xbsIndex_r4/Constant  const=0  gui_display_data_type=Fixed-point  arith_type=Boolean  n_bits=32  bin_pt=0  preci_type=Single  exp_width=8  frac_width=24  explicit_period=off  period=1  equ=P=C  opselect=C  inp2=PCIN>>17  opr=+  inp1=P  carry=CIN  dbl_ovrd=off  block_type=constant
      settings: block_version=10.1.2
  Constant2 : xbsIndex_r4/Constant  const=0  gui_display_data_type=Fixed-point  arith_type=Unsigned  n_bits=32  bin_pt=0  preci_type=Single  exp_width=8  frac_width=24  explicit_period=off  period=1  equ=P=C  opselect=C  inp2=PCIN>>17  opr=+  inp1=P  carry=CIN  dbl_ovrd=off  block_type=constant
      settings: block_version=10.1.2
  Shared Memory : xbsIndex_r4/Shared Memory  shared_memory_name='RFD_IQ_Rx_Buffer'  depth=NumSamps_Rx_IQ  ownership=Locally Owned and Initialized  initVector=0  en=off  mutex=Unprotected  mode=Read and Write  write_mode=Read After Write  time_out=0  latency=1  explicit_data_type=on  gui_display_data_type=Fixed-point  arith_type=Unsigned  n_bits=32  bin_pt=0  preci_type=Single  implementation=Block RAM  use_rpm=off  block_type=shmem
      settings: AttributesFormatString=<< %<shared_memory_name> >>  block_version=10.1.2
  Shared Memory1 : xbsIndex_r4/Shared Memory  shared_memory_name='RFD_RSSI_Buffer'  depth=NumSamps_Rx_RSSI/2  ownership=Locally Owned and Initialized  initVector=0  en=off  mutex=Unprotected  mode=Read and Write  write_mode=Read After Write  time_out=0  latency=1  explicit_data_type=on  gui_display_data_type=Fixed-point  arith_type=Unsigned  n_bits=32  bin_pt=0  preci_type=Single  implementation=Block RAM  use_rpm=off  block_type=shmem
      settings: AttributesFormatString=<< %<shared_memory_name> >>  block_version=10.1.2
  Shared Memory2 : xbsIndex_r4/Shared Memory  shared_memory_name='RFD_IQ_Tx_Buffer'  depth=NumSamps_Tx_IQ  ownership=Locally Owned and Initialized  initVector=0  en=off  mutex=Unprotected  mode=Read and Write  write_mode=Read After Write  time_out=0  latency=1  explicit_data_type=on  gui_display_data_type=Fixed-point  arith_type=Unsigned  n_bits=32  bin_pt=0  preci_type=Single  implementation=Block RAM  use_rpm=off  block_type=shmem
      settings: AttributesFormatString=<< %<shared_memory_name> >>  block_version=10.1.2
  Terminator : Terminator
  Terminator2 : Terminator
  b[13:0] : xbsIndex_r4/Slice  nbits=14  boolean_output=off  mode=Lower Bit Location + Width  bit1=0  base1=MSB of Input  bit0=0  base0=LSB of Input  dbl_ovrd=off  block_type=slice
  rx_addr[13:0] : xbsIndex_r4/Slice  nbits=14  boolean_output=off  mode=Lower Bit Location + Width  bit1=0  base1=MSB of Input  bit0=0  base0=LSB of Input  dbl_ovrd=off  block_type=slice
  IQ_TX_DOUT : Outport
  tag scope: RFD_IQ_RX_ADDR_SCOPE=global, RFD_IQ_RX_DOUT_SCOPE=global, RFD_IQ_RX_WEN_SCOPE=global, RFD_IQ_TX_ADDR_SCOPE=global, RFD_IQ_TX_DOUT_RAW_SCOPE=global, RFD_IQ_TX_DOUT_SCOPE=global, RFD_IQ_TX_SEL_SCOPE=global
  wires:
  IQ_RX_WEN/1 -> Shared Memory/3, [RFD_IQ_RX_WEN_SCOPE], [RFD_IQ_RX_DOUT_SCOPE]
  IQ_RX_ADDR/1 -> rx_addr[13:0]/1
  Shared Memory/1 -> Terminator/1
  IQ_RX_DIN/1 -> Shared Memory/2
  Shared Memory1/1 -> Terminator2/1
  RSSI_ADDR/1 -> Shared Memory1/1
  RSSI_DIN/1 -> Shared Memory1/2
  RSSI_WEN/1 -> Shared Memory1/3
  IQ_TX_ADDR/1 -> [RFD_IQ_TX_ADDR_SCOPE], b[13:0]/1
  Constant1/1 -> Shared Memory2/3, [RFD_IQ_TX_SEL_SCOPE]
  Constant2/1 -> Shared Memory2/2
  Shared Memory2/1 -> IQ_TX_DOUT/1, [RFD_IQ_TX_DOUT_RAW_SCOPE], [RFD_IQ_TX_DOUT_SCOPE]
  b[13:0]/1 -> Shared Memory2/1
  rx_addr[13:0]/1 -> Shared Memory/1, [RFD_IQ_RX_ADDR_SCOPE]

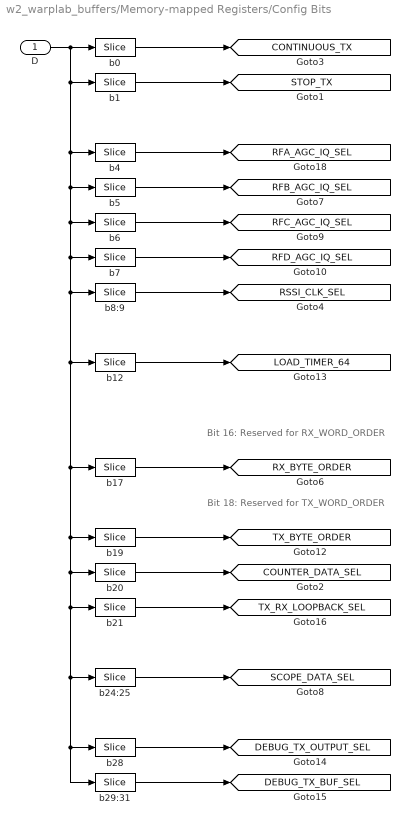
== system w2_warplab_buffers/Memory-mapped Registers/Config Bits ==
  note: Bit 16: Reserved for RX_WORD_ORDER
  note: Bit 18: Reserved for TX_WORD_ORDER
  D : Inport
  b0 : xbsIndex_r4/Slice  nbits=1  boolean_output=off  mode=Lower Bit Location + Width  bit1=0  base1=MSB of Input  bit0=0  base0=LSB of Input  dbl_ovrd=off  block_type=slice
  b1 : xbsIndex_r4/Slice  nbits=1  boolean_output=off  mode=Lower Bit Location + Width  bit1=0  base1=MSB of Input  bit0=1  base0=LSB of Input  dbl_ovrd=off  block_type=slice
  b12 : xbsIndex_r4/Slice  nbits=1  boolean_output=off  mode=Lower Bit Location + Width  bit1=0  base1=MSB of Input  bit0=12  base0=LSB of Input  dbl_ovrd=off  block_type=slice
  b17 : xbsIndex_r4/Slice  nbits=1  boolean_output=off  mode=Lower Bit Location + Width  bit1=0  base1=MSB of Input  bit0=17  base0=LSB of Input  dbl_ovrd=off  block_type=slice
  b19 : xbsIndex_r4/Slice  nbits=1  boolean_output=off  mode=Lower Bit Location + Width  bit1=0  base1=MSB of Input  bit0=19  base0=LSB of Input  dbl_ovrd=off  block_type=slice
  b20 : xbsIndex_r4/Slice  nbits=1  boolean_output=off  mode=Lower Bit Location + Width  bit1=0  base1=MSB of Input  bit0=20  base0=LSB of Input  dbl_ovrd=off  block_type=slice
  b21 : xbsIndex_r4/Slice  nbits=1  boolean_output=off  mode=Lower Bit Location + Width  bit1=0  base1=MSB of Input  bit0=21  base0=LSB of Input  dbl_ovrd=off  block_type=slice
  b24:25 : xbsIndex_r4/Slice  nbits=2  boolean_output=off  mode=Lower Bit Location + Width  bit1=0  base1=MSB of Input  bit0=24  base0=LSB of Input  dbl_ovrd=off  block_type=slice
  b28 : xbsIndex_r4/Slice  nbits=1  boolean_output=off  mode=Lower Bit Location + Width  bit1=0  base1=MSB of Input  bit0=28  base0=LSB of Input  dbl_ovrd=off  block_type=slice
  b29:31 : xbsIndex_r4/Slice  nbits=3  boolean_output=off  mode=Lower Bit Location + Width  bit1=0  base1=MSB of Input  bit0=29  base0=LSB of Input  dbl_ovrd=off  block_type=slice
  b4 : xbsIndex_r4/Slice  nbits=1  boolean_output=off  mode=Lower Bit Location + Width  bit1=0  base1=MSB of Input  bit0=4  base0=LSB of Input  dbl_ovrd=off  block_type=slice
  b5 : xbsIndex_r4/Slice  nbits=1  boolean_output=off  mode=Lower Bit Location + Width  bit1=0  base1=MSB of Input  bit0=5  base0=LSB of Input  dbl_ovrd=off  block_type=slice
  b6 : xbsIndex_r4/Slice  nbits=1  boolean_output=off  mode=Lower Bit Location + Width  bit1=0  base1=MSB of Input  bit0=6  base0=LSB of Input  dbl_ovrd=off  block_type=slice
  b7 : xbsIndex_r4/Slice  nbits=1  boolean_output=off  mode=Lower Bit Location + Width  bit1=0  base1=MSB of Input  bit0=7  base0=LSB of Input  dbl_ovrd=off  block_type=slice
  b8:9 : xbsIndex_r4/Slice  nbits=2  boolean_output=off  mode=Lower Bit Location + Width  bit1=0  base1=MSB of Input  bit0=8  base0=LSB of Input  dbl_ovrd=off  block_type=slice
  tag scope: CONTINUOUS_TX=global, COUNTER_DATA_SEL=global, DEBUG_TX_BUF_SEL=global, DEBUG_TX_OUTPUT_SEL=global, LOAD_TIMER_64=global, RFA_AGC_IQ_SEL=global, RFB_AGC_IQ_SEL=global, RFC_AGC_IQ_SEL=global, RFD_AGC_IQ_SEL=global, RSSI_CLK_SEL=global, RX_BYTE_ORDER=global, SCOPE_DATA_SEL=global, STOP_TX=global, TX_BYTE_ORDER=global, TX_RX_LOOPBACK_SEL=global
  wires:
  D/1 -> b1/1, b4/1, b5/1, b6/1, b7/1, b17/1, b8:9/1, b12/1, b20/1, b24:25/1, b28/1, b29:31/1, b21/1, b19/1, b0/1
  b0/1 -> [CONTINUOUS_TX]
  b1/1 -> [STOP_TX]
  b4/1 -> [RFA_AGC_IQ_SEL]
  b17/1 -> [RX_BYTE_ORDER]
  b8:9/1 -> [RSSI_CLK_SEL]
  b20/1 -> [COUNTER_DATA_SEL]
  b24:25/1 -> [SCOPE_DATA_SEL]
  b5/1 -> [RFB_AGC_IQ_SEL]
  b6/1 -> [RFC_AGC_IQ_SEL]
  b7/1 -> [RFD_AGC_IQ_SEL]
  b19/1 -> [TX_BYTE_ORDER]
  b12/1 -> [LOAD_TIMER_64]
  b28/1 -> [DEBUG_TX_OUTPUT_SEL]
  b29:31/1 -> [DEBUG_TX_BUF_SEL]
  b21/1 -> [TX_RX_LOOPBACK_SEL]

== system w2_warplab_buffers/Memory-mapped Registers/RFx Sel ==
  32b : Inport
  b0 : xbsIndex_r4/Slice  nbits=1  boolean_output=off  mode=Lower Bit Location + Width  bit1=0  base1=MSB of Input  bit0=0  base0=LSB of Input  dbl_ovrd=off  block_type=slice
  b1 : xbsIndex_r4/Slice  nbits=1  boolean_output=off  mode=Lower Bit Location + Width  bit1=0  base1=MSB of Input  bit0=1  base0=LSB of Input  dbl_ovrd=off  block_type=slice
  b2 : xbsIndex_r4/Slice  nbits=1  boolean_output=off  mode=Lower Bit Location + Width  bit1=1  base1=MSB of Input  bit0=2  base0=LSB of Input  dbl_ovrd=off  block_type=slice
  b3 : xbsIndex_r4/Slice  nbits=1  boolean_output=off  mode=Lower Bit Location + Width  bit1=1  base1=MSB of Input  bit0=3  base0=LSB of Input  dbl_ovrd=off  block_type=slice
  A : Outport
  B : Outport  Port=2
  C : Outport  Port=3
  D : Outport  Port=4
  wires:
  32b/1 -> b0/1, b1/1, b2/1, b3/1
  b3/1 -> D/1
  b2/1 -> C/1
  b1/1 -> B/1
  b0/1 -> A/1

== system w2_warplab_buffers/Memory-mapped Registers/RFx Sel2 ==
  32b : Inport
  b0 : xbsIndex_r4/Slice  nbits=1  boolean_output=off  mode=Lower Bit Location + Width  bit1=0  base1=MSB of Input  bit0=0  base0=LSB of Input  dbl_ovrd=off  block_type=slice
  b1 : xbsIndex_r4/Slice  nbits=1  boolean_output=off  mode=Lower Bit Location + Width  bit1=0  base1=MSB of Input  bit0=1  base0=LSB of Input  dbl_ovrd=off  block_type=slice
  b2 : xbsIndex_r4/Slice  nbits=1  boolean_output=off  mode=Lower Bit Location + Width  bit1=1  base1=MSB of Input  bit0=2  base0=LSB of Input  dbl_ovrd=off  block_type=slice
  b3 : xbsIndex_r4/Slice  nbits=1  boolean_output=off  mode=Lower Bit Location + Width  bit1=1  base1=MSB of Input  bit0=3  base0=LSB of Input  dbl_ovrd=off  block_type=slice
  A : Outport
  B : Outport  Port=2
  C : Outport  Port=3
  D : Outport  Port=4
  wires:
  32b/1 -> b0/1, b1/1, b2/1, b3/1
  b3/1 -> D/1
  b2/1 -> C/1
  b1/1 -> B/1
  b0/1 -> A/1

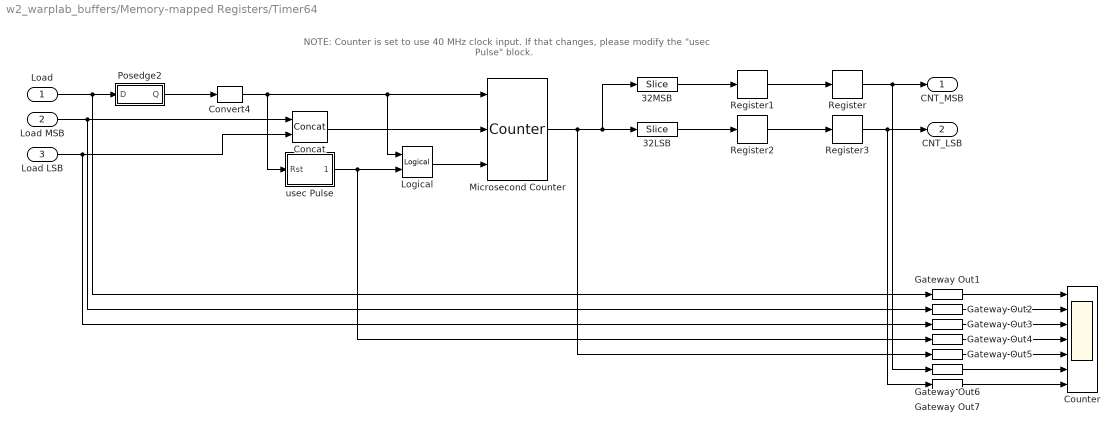
== system w2_warplab_buffers/Memory-mapped Registers/Timer64 ==
  note: NOTE: Counter is set to use 40 MHz clock input. If that changes, please modify the "usec Pulse" block.
  Load : Inport
  Load MSB : Inport  Port=2
  Load LSB : Inport  Port=3
  32LSB : xbsIndex_r4/Slice  nbits=32  boolean_output=off  mode=Lower Bit Location + Width  bit1=0  base1=MSB of Input  bit0=0  base0=LSB of Input  dbl_ovrd=off  block_type=slice
      settings: block_version=VER_STRING_GOES_HERE
  32MSB : xbsIndex_r4/Slice  nbits=32  boolean_output=off  mode=Upper Bit Location + Width  bit1=0  base1=MSB of Input  bit0=0  base0=LSB of Input  dbl_ovrd=off  block_type=slice
      settings: block_version=VER_STRING_GOES_HERE
  Concat : xbsIndex_r4/Concat  num_inputs=2  dbl_ovrd=off  block_type=concat
  Convert4 : xbsIndex_r4/Convert  gui_display_data_type=Boolean  arith_type=Boolean  n_bits=32  bin_pt=0  float_type=Single  exp_bits=8  fraction_bits=24  quantization=Truncate  overflow=Wrap  en=off  latency=0  dbl_ovrd=off  pipeline=off  block_type=convert
      settings: block_version=8.2
  Counter : Scope  NumInputPorts=7
      settings: TimeRange=70000  YMin=0~0~0~0~0~-5~-5  YMax=1~1~1~100~20000~5~5  SaveName=ScopeData7
  Gateway Out{1..7} (7 alike) : xbsIndex_r4/Gateway Out  inherit_from_input=off  hdl_port=off  timing_constraint=None  locs_specified=off  LOCs={}  UseAsDAC=off  DACChannel='1'  block_type=gatewayout
      settings: infoedit="Gateway out block.  Converts Xilinx fixed point inputs into ouputs of type Simulink integer, double, or fixed point.<P><P>Hardware notes:  In hardware these blocks become top level output ports or are discarded, depending on how they are configured."  block_version=10.1.2
  Logical : xbsIndex_r4/Logical  logical_function=OR  inputs=2  en=off  latency=0  precision=Full  arith_type=Unsigned  n_bits=16  bin_pt=0  align_bp=on  dbl_ovrd=off  block_type=logical
  Microsecond Counter : xbsIndex_r4/Counter  cnt_type=Free Running  cnt_to=Inf  operation=Up  start_count=0  cnt_by_val=1  arith_type=Unsigned  n_bits=64  bin_pt=0  load_pin=on  rst=off  en=on  explicit_period=off  period=1  dbl_ovrd=off  use_behavioral_HDL=off  implementation=Fabric  block_type=counter
  Posedge2 : Subsystem
  Register{,1..3} (4 alike) : xbsIndex_r4/Register  init=0  rst=off  en=off  dbl_ovrd=off  block_type=register
  usec Pulse : Subsystem
  CNT_MSB : Outport
  CNT_LSB : Outport  Port=2
  wires:
  Microsecond Counter/1 -> 32LSB/1, 32MSB/1, Gateway Out5/1
  32LSB/1 -> Register2/1
  32MSB/1 -> Register1/1
  Register/1 -> CNT_MSB/1, Gateway Out6/1
  Register1/1 -> Register/1
  Register2/1 -> Register3/1
  Register3/1 -> CNT_LSB/1, Gateway Out7/1
  Logical/1 -> Microsecond Counter/3
  usec Pulse/1(uSec) -> Logical/2, Gateway Out4/1
  Load LSB/1 -> Concat/2, Gateway Out3/1
  Load MSB/1 -> Concat/1, Gateway Out2/1
  Concat/1 -> Microsecond Counter/2
  Load/1 -> Posedge2/1(D), Gateway Out1/1
  Posedge2/1(Q) -> Convert4/1
  Convert4/1 -> Microsecond Counter/1, Logical/1, usec Pulse/1(Rst)
  Gateway Out5/1 -> Counter/5
  Gateway Out4/1 -> Counter/4
  Gateway Out3/1 -> Counter/3
  Gateway Out2/1 -> Counter/2
  Gateway Out1/1 -> Counter/1
  Gateway Out7/1 -> Counter/7
  Gateway Out6/1 -> Counter/6
